simulink model "Boeing787_NewMission_ElectricalThermalHydraulicECS"  (R2016a)
settings: Solver=ode23tb  SolverMode=SingleTasking  StartTime=0.0  StopTime=346  RelTol=1e-3
InitFcn:
  | load('SampleOutput.mat')
  | 
  | load('SampleFuelBurn.mat')
undefined symbols (not defined in the file): ailerons, AirProp, B_737, CurrentMission, elevator, FuelBurn, HydProp, landing_gear, rudder, seed, thrust_rev
libraries: PowerFlowLib x68, simulink x20, powerlib_meascontrol x1
(part 15 of 24)

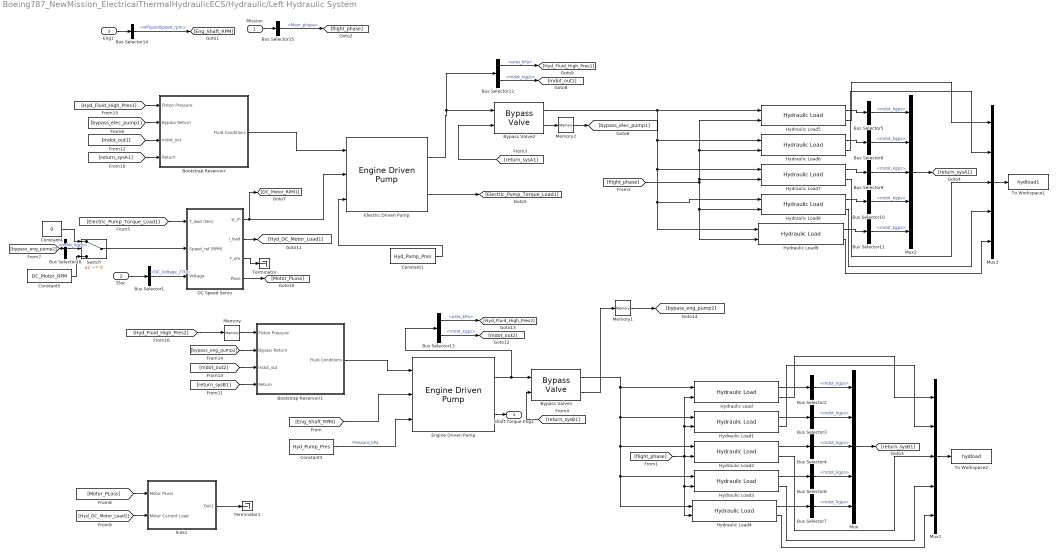
== system Boeing787_NewMission_ElectricalThermalHydraulicECS/Hydraulic/Left Hydraulic System ==
  Mission : Inport
  Elec : Inport  Port=2
  Eng1 : Inport  Port=3
  Bootstrap Reservoir : Subsystem  mask(Fluid Reservoir){res_vol=.25, High_Pres_Area=.05, Low_Pres_Area=0, pres_loss=1, T_init=300, P_init=1500, mass_init=30}
      mask prompts: res_vol "Resevoir Volume [m³]"; High_Pres_Area "High Pressure Piston Area"; Low_Pres_Area "Low Pressure Piston Area"; pres_loss "Air Pressure Losses [%]"; T_init "Initial Fluid Temp [K]"; P_init "Initial Air Pressure [kPa]"; mass_init "Initial Fluid Mass [kg]"
      mask help:
      | The fluid reservoir serves as a tank for storing excess hydraulic fluid.
      | The reservoir is fed by returning hydraulic fluid and feeds the engine driven pump.
      | Currently the fluid reservoir tracks the time dependent mass and temperature of the hydraulic fluid in the tank.
      |
      | Block Inputs
      | #1: Bleed air properties (Bus signal)
      | #2: Bypass return from bypass valve
      | #3: Mass flow rate pumped out by hydraulic pump
      | #4: Mass flow rate returned from actuators
      |
      | Block Outputs
      | #1: Bleed air demanded to maintain pressurization
      | #2: Hydraulic fluid properties in the reservoir
      mask init:
      | load AirProp
      | load HydProp
      mask Help: eval('open(''FluidReservoir_help.html'')');
      mask Display:
      | image(imread('hyd_res.png'))
      | 
      | port_label('input',1,'{\bf High Piston Pressure}','TexMode','on')
      | port_label('input',2,'{\bf Bypass Return}','TexMode','on')
      | port_label('input',3,'{\bf m_d_o_t Out}','TexMode','on')
      | port_label('input',4,'{\bf m_d_o_t Return}','TexMode','on')
      | 
      | 
      | port_label('output',1,'{\bf Fluid Out}','TexMode','on')
  Bootstrap Reservoir1 : Subsystem  mask(Fluid Reservoir){res_vol=.25, High_Pres_Area=.05, Low_Pres_Area=0, pres_loss=1, T_init=300, P_init=1500, mass_init=30}
      mask prompts: res_vol "Resevoir Volume [m³]"; High_Pres_Area "High Pressure Piston Area"; Low_Pres_Area "Low Pressure Piston Area"; pres_loss "Air Pressure Losses [%]"; T_init "Initial Fluid Temp [K]"; P_init "Initial Air Pressure [kPa]"; mass_init "Initial Fluid Mass [kg]"
      mask help:
      | The fluid reservoir serves as a tank for storing excess hydraulic fluid.
      | The reservoir is fed by returning hydraulic fluid and feeds the engine driven pump.
      | Currently the fluid reservoir tracks the time dependent mass and temperature of the hydraulic fluid in the tank.
      |
      | Block Inputs
      | #1: Bleed air properties (Bus signal)
      | #2: Bypass return from bypass valve
      | #3: Mass flow rate pumped out by hydraulic pump
      | #4: Mass flow rate returned from actuators
      |
      | Block Outputs
      | #1: Bleed air demanded to maintain pressurization
      | #2: Hydraulic fluid properties in the reservoir
      mask init:
      | load AirProp
      | load HydProp
      mask Help: eval('open(''FluidReservoir_help.html'')');
      mask Display:
      | image(imread('hyd_res.png'))
      | 
      | port_label('input',1,'{\bf High Piston Pressure}','TexMode','on')
      | port_label('input',2,'{\bf Bypass Return}','TexMode','on')
      | port_label('input',3,'{\bf m_d_o_t Out}','TexMode','on')
      | port_label('input',4,'{\bf m_d_o_t Return}','TexMode','on')
      | 
      | 
      | port_label('output',1,'{\bf Fluid Out}','TexMode','on')
  Bus Selector1 : BusSelector  OutputSignals=signal1.DC_Voltage_270
  Bus Selector{2..11,16} (11 alike) : BusSelector  OutputSignals=mdot_kgps
  Bus Selector12 : BusSelector  OutputSignals=pres_kPa,mdot_kgps
  Bus Selector13 : BusSelector  OutputSignals=pres_kPa,mdot_kgps
  Bus Selector14 : BusSelector  OutputSignals=Spools.HPSpoolSpeed_rpm
  Bus Selector15 : BusSelector  OutputSignals=Mssn_phase
  Bypass Valve1 : PowerFlowLib/Energy & Power Systems/Hydraulic/Bypass Valve
  Bypass Valve2 : PowerFlowLib/Energy & Power Systems/Hydraulic/Bypass Valve
  Constant1 : Constant  Value=Hyd_Pump_Pres
  Constant3 : Constant  Value=Hyd_Pump_Pres
  Constant4 : Constant  Value=0
  Constant5 : Constant  Value=DC_Motor_RPM
  DC Speed Servo : Subsystem  AncestorBlock=PowerFlowLib/Energy & Power Systems/Electrical/Machines/DC Speed Servo  mask{Vf=280, Ra=0.05, La=0.9e-3, Rfsh=400, Lfsh=320, Lmsh=1.9, J=1.5}
      mask prompts: Vf "Field voltage (V)"; Ra "Armature resistance (Ohms)"; La "Armature inductance (H)"; Rfsh "Shunt field resistance (Ohms)"; Lfsh "Shunt field inductance (H)"; Lmsh "Mutual inductance (H)"; J "Rotor moment of inertia (Kgm^2)"
  Electric Driven Pump : PowerFlowLib/Energy & Power Systems/Hydraulic/Engine Driven Pump  RPM=3750  disp=39  eta_mech=95  eta_v=85  nom_T=40  nom_w=393  nom_delP=20684
  Engine Driven Pump : PowerFlowLib/Energy & Power Systems/Hydraulic/Engine Driven Pump  RPM=3750  disp=39  eta_mech=95  eta_v=85  nom_T=40  nom_w=393  nom_delP=20684
  Hydraulic Load : PowerFlowLib/Energy & Power Systems/Hydraulic/Hydraulic Load  fileslct=off  filename=HydraulicLoad.mat  filedir=C:\Users\mwillms4\Dropbox\School\Graduate\Research\PowerFlow Development\PowerFlow Summer 2013\PropertyTables\HydraulicLoad.mat  var_struct=HydraulicLoad  h_load=B_737 - rudder
  Hydraulic Load1 : PowerFlowLib/Energy & Power Systems/Hydraulic/Hydraulic Load  fileslct=off  filename=HydraulicLoad.mat  filedir=C:\Users\mwillms4\Dropbox\School\Graduate\Research\PowerFlow Development\PowerFlow Summer 2013\PropertyTables\HydraulicLoad.mat  var_struct=HydraulicLoad  h_load=B_737 - ailerons
  Hydraulic Load2 : PowerFlowLib/Energy & Power Systems/Hydraulic/Hydraulic Load  fileslct=off  filename=HydraulicLoad.mat  filedir=C:\Users\mwillms4\Dropbox\School\Graduate\Research\PowerFlow Development\PowerFlow Summer 2013\PropertyTables\HydraulicLoad.mat  var_struct=HydraulicLoad  h_load=B_737 - elevator
  Hydraulic Load3 : PowerFlowLib/Energy & Power Systems/Hydraulic/Hydraulic Load  fileslct=off  filename=HydraulicLoad.mat  filedir=C:\Users\mwillms4\Dropbox\School\Graduate\Research\PowerFlow Development\PowerFlow Summer 2013\PropertyTables\HydraulicLoad.mat  var_struct=HydraulicLoad  h_load=B_737 - landing_gear
  Hydraulic Load4 : PowerFlowLib/Energy & Power Systems/Hydraulic/Hydraulic Load  fileslct=off  filename=HydraulicLoad.mat  filedir=C:\Users\mwillms4\Dropbox\School\Graduate\Research\PowerFlow Development\PowerFlow Summer 2013\PropertyTables\HydraulicLoad.mat  var_struct=HydraulicLoad  h_load=B_737 - thrust_rev
  Hydraulic Load5 : PowerFlowLib/Energy & Power Systems/Hydraulic/Hydraulic Load  fileslct=off  filename=HydraulicLoad.mat  filedir=C:\Users\mwillms4\Dropbox\School\Graduate\Research\PowerFlow Development\PowerFlow Summer 2013\PropertyTables\HydraulicLoad.mat  var_struct=HydraulicLoad  h_load=B_737 - rudder
  Hydraulic Load6 : PowerFlowLib/Energy & Power Systems/Hydraulic/Hydraulic Load  fileslct=off  filename=HydraulicLoad.mat  filedir=C:\Users\mwillms4\Dropbox\School\Graduate\Research\PowerFlow Development\PowerFlow Summer 2013\PropertyTables\HydraulicLoad.mat  var_struct=HydraulicLoad  h_load=B_737 - ailerons
  Hydraulic Load7 : PowerFlowLib/Energy & Power Systems/Hydraulic/Hydraulic Load  fileslct=off  filename=HydraulicLoad.mat  filedir=C:\Users\mwillms4\Dropbox\School\Graduate\Research\PowerFlow Development\PowerFlow Summer 2013\PropertyTables\HydraulicLoad.mat  var_struct=HydraulicLoad  h_load=B_737 - elevator
  Hydraulic Load8 : PowerFlowLib/Energy & Power Systems/Hydraulic/Hydraulic Load  fileslct=off  filename=HydraulicLoad.mat  filedir=C:\Users\mwillms4\Dropbox\School\Graduate\Research\PowerFlow Development\PowerFlow Summer 2013\PropertyTables\HydraulicLoad.mat  var_struct=HydraulicLoad  h_load=B_737 - landing_gear
  Hydraulic Load9 : PowerFlowLib/Energy & Power Systems/Hydraulic/Hydraulic Load  fileslct=off  filename=HydraulicLoad.mat  filedir=C:\Users\mwillms4\Dropbox\School\Graduate\Research\PowerFlow Development\PowerFlow Summer 2013\PropertyTables\HydraulicLoad.mat  var_struct=HydraulicLoad  h_load=B_737 - thrust_rev
  Memory : Memory
  Memory1 : Memory
  Memory2 : Memory
  Mux{,1..3} (4 alike) : Mux  Inputs=5
  Sinks : Subsystem
  Switch : Switch  Criteria=u2 ~= 0
  Terminator : Terminator
  Terminator1 : Terminator
  To Workspace1 : ToWorkspace  VariableName=hydload1  SaveFormat=Structure With Time  SampleTime=10
  To Workspace2 : ToWorkspace  VariableName=hydload  SaveFormat=Structure With Time  SampleTime=10
  Shaft Torque Eng1 : Outport
  wires:
  Bus Selector15/1 -> [flight_phase]  "<Mssn_phase>"
  Mission/1 -> Bus Selector15/1
  DC Speed Servo/1(w_m) -> Electric Driven Pump/2, [DC_Motor_RPM1]
  Constant3/1 -> Engine Driven Pump/3  "Pressure_kPa"
  Eng1/1 -> Bus Selector14/1
  [Eng_Shaft_RPM] -> Engine Driven Pump/2
  Elec/1 -> Bus Selector1/1
  Bus Selector1/1 -> DC Speed Servo/3(Voltage)  "<DC_Voltage_270>"
  Engine Driven Pump/2 -> Shaft Torque Eng1/1
  Hydraulic Load/1 -> Bus Selector2/1
  Bypass Valve1/1 -> Hydraulic Load3/1, Hydraulic Load4/1, Hydraulic Load2/1, Hydraulic Load1/1, Hydraulic Load/1
  Hydraulic Load1/2 -> Mux1/2
  Hydraulic Load2/2 -> Mux1/3
  Hydraulic Load1/1 -> Bus Selector3/1
  Hydraulic Load2/1 -> Bus Selector4/1
  Bus Selector3/1 -> Mux/2  "<mdot_kgps>"
  Bus Selector2/1 -> Mux/1  "<mdot_kgps>"
  Bus Selector4/1 -> Mux/3  "<mdot_kgps>"
  Mux/1 -> [return_sysB1]
  [flight_phase] -> Hydraulic Load/2, Hydraulic Load1/2, Hydraulic Load3/2, Hydraulic Load4/2, Hydraulic Load2/2
  Hydraulic Load3/1 -> Bus Selector6/1
  Hydraulic Load4/1 -> Bus Selector7/1
  Hydraulic Load4/2 -> Mux1/5
  Hydraulic Load3/2 -> Mux1/4
  Bus Selector6/1 -> Mux/4  "<mdot_kgps>"
  Bus Selector7/1 -> Mux/5  "<mdot_kgps>"
  Hydraulic Load/2 -> Mux1/1
  Mux1/1 -> To Workspace2/1
  Hydraulic Load5/1 -> Bus Selector5/1
  Bypass Valve2/1 -> Hydraulic Load9/1, Hydraulic Load8/1, Hydraulic Load7/1, Hydraulic Load6/1, Hydraulic Load5/1
  Hydraulic Load6/2 -> Mux3/2
  Hydraulic Load7/2 -> Mux3/3
  Hydraulic Load6/1 -> Bus Selector8/1
  Hydraulic Load7/1 -> Bus Selector9/1
  Bus Selector8/1 -> Mux2/2  "<mdot_kgps>"
  Bus Selector5/1 -> Mux2/1  "<mdot_kgps>"
  Bus Selector9/1 -> Mux2/3  "<mdot_kgps>"
  Mux2/1 -> [return_sysA1]
  [flight_phase] -> Hydraulic Load9/2, Hydraulic Load8/2, Hydraulic Load5/2, Hydraulic Load6/2, Hydraulic Load7/2
  Hydraulic Load8/1 -> Bus Selector10/1
  Hydraulic Load9/1 -> Bus Selector11/1
  Hydraulic Load9/2 -> Mux3/5
  Hydraulic Load8/2 -> Mux3/4
  Bus Selector10/1 -> Mux2/4  "<mdot_kgps>"
  Bus Selector11/1 -> Mux2/5  "<mdot_kgps>"
  Hydraulic Load5/2 -> Mux3/1
  Mux3/1 -> To Workspace1/1
  Engine Driven Pump/1 -> Bus Selector13/1, Bypass Valve1/1
  Electric Driven Pump/1 -> Bus Selector12/1, Bypass Valve2/1
  [return_sysA1] -> Bypass Valve2/2
  [return_sysB1] -> Bypass Valve1/2
  Constant1/1 -> Electric Driven Pump/3
  Electric Driven Pump/2 -> [Electric_Pump_Torque_Load1]
  [Electric_Pump_Torque_Load1] -> DC Speed Servo/1(T_load (Nm))
  Bypass Valve2/2 -> Memory2/1
  [bypass_elec_pump1] -> Bootstrap Reservoir/2(Bypass Return)
  Bootstrap Reservoir/1(Fluid Conditions) -> Electric Driven Pump/1
  Constant4/1 -> Switch/1
  Bus Selector12/1 -> [Hyd_Fluid_High_Pres1]  "<pres_kPa>"
  Bus Selector12/2 -> [mdot_out1]  "<mdot_kgps>"
  DC Speed Servo/4(Ploss) -> [Motor_PLoss]
  [Motor_PLoss] -> Sinks/1("Motor PLoss ")
  DC Speed Servo/2(i_load) -> [Hyd_DC_Motor_Load1]
  [Hyd_DC_Motor_Load1] -> Sinks/2(Motor Current Load)
  Bootstrap Reservoir1/1(Fluid Conditions) -> Engine Driven Pump/1
  Bus Selector13/1 -> [Hyd_Fluid_High_Pres2]  "<pres_kPa>"
  Bus Selector13/2 -> [mdot_out2]  "<mdot_kgps>"
  [return_sysA1] -> Bootstrap Reservoir/4(Return)
  [return_sysB1] -> Bootstrap Reservoir1/4(Return)
  [mdot_out1] -> Bootstrap Reservoir/3(mdot_out)
  Bypass Valve1/2 -> Memory1/1
  [bypass_eng_pump2] -> Bootstrap Reservoir1/2(Bypass Return)
  [mdot_out2] -> Bootstrap Reservoir1/3(mdot_out)
  [Hyd_Fluid_High_Pres1] -> Bootstrap Reservoir/1(Piston Pressure)
  [Hyd_Fluid_High_Pres2] -> Memory/1
  Bus Selector14/1 -> [Eng_Shaft_RPM]  "<HPSpoolSpeed_rpm>"
  DC Speed Servo/3(T_em) -> Terminator/1
  Sinks/1(Out1) -> Terminator1/1
  Memory/1 -> Bootstrap Reservoir1/1(Piston Pressure)
  [bypass_eng_pump2] -> Bus Selector16/1
  Constant5/1 -> Switch/3
  Bus Selector16/1 -> Switch/2  "<mdot_kgps>"
  Switch/1 -> DC Speed Servo/2(Speed_ref (RPM))
  Memory1/1 -> [bypass_eng_pump2]
  Memory2/1 -> [bypass_elec_pump1]

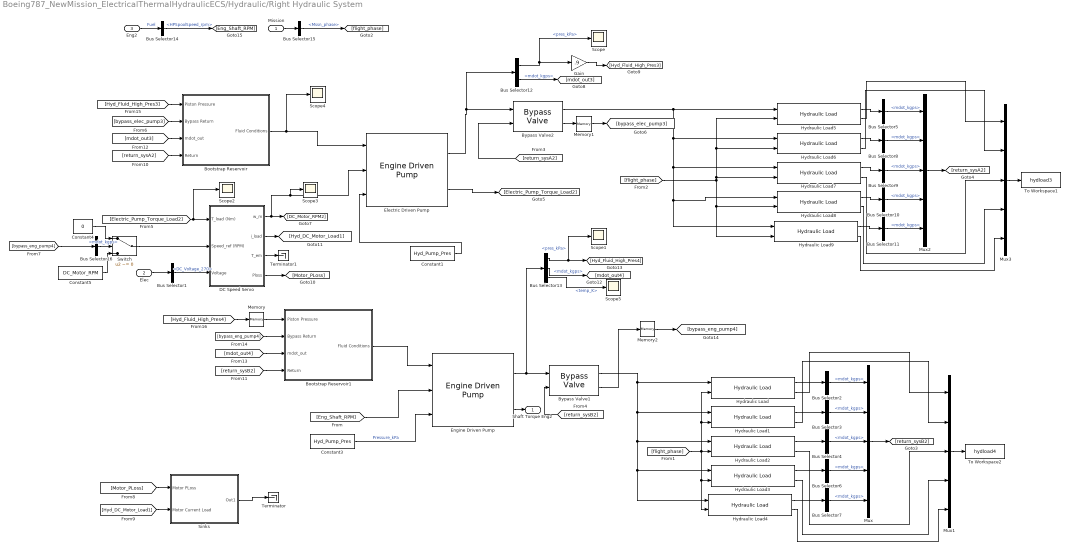
== system Boeing787_NewMission_ElectricalThermalHydraulicECS/Hydraulic/Right Hydraulic System ==
  Mission : Inport
  Elec : Inport  Port=2
  Eng2 : Inport  Port=3
  Bootstrap Reservoir : Subsystem  mask(Fluid Reservoir){res_vol=.25, High_Pres_Area=.05, Low_Pres_Area=0, pres_loss=1, T_init=300, P_init=1500, mass_init=30}
      mask prompts: res_vol "Resevoir Volume [m³]"; High_Pres_Area "High Pressure Piston Area"; Low_Pres_Area "Low Pressure Piston Area"; pres_loss "Air Pressure Losses [%]"; T_init "Initial Fluid Temp [K]"; P_init "Initial Air Pressure [kPa]"; mass_init "Initial Fluid Mass [kg]"
      mask help:
      | The fluid reservoir serves as a tank for storing excess hydraulic fluid.
      | The reservoir is fed by returning hydraulic fluid and feeds the engine driven pump.
      | Currently the fluid reservoir tracks the time dependent mass and temperature of the hydraulic fluid in the tank.
      |
      | Block Inputs
      | #1: Bleed air properties (Bus signal)
      | #2: Bypass return from bypass valve
      | #3: Mass flow rate pumped out by hydraulic pump
      | #4: Mass flow rate returned from actuators
      |
      | Block Outputs
      | #1: Bleed air demanded to maintain pressurization
      | #2: Hydraulic fluid properties in the reservoir
      mask init:
      | load AirProp
      | load HydProp
      mask Help: eval('open(''FluidReservoir_help.html'')');
      mask Display:
      | image(imread('hyd_res.png'))
      | 
      | port_label('input',1,'{\bf High Piston Pressure}','TexMode','on')
      | port_label('input',2,'{\bf Bypass Return}','TexMode','on')
      | port_label('input',3,'{\bf m_d_o_t Out}','TexMode','on')
      | port_label('input',4,'{\bf m_d_o_t Return}','TexMode','on')
      | 
      | 
      | port_label('output',1,'{\bf Fluid Out}','TexMode','on')
  Bootstrap Reservoir1 : Subsystem  mask(Fluid Reservoir){res_vol=.25, High_Pres_Area=.05, Low_Pres_Area=0, pres_loss=1, T_init=300, P_init=1500, mass_init=30}
      mask prompts: res_vol "Resevoir Volume [m³]"; High_Pres_Area "High Pressure Piston Area"; Low_Pres_Area "Low Pressure Piston Area"; pres_loss "Air Pressure Losses [%]"; T_init "Initial Fluid Temp [K]"; P_init "Initial Air Pressure [kPa]"; mass_init "Initial Fluid Mass [kg]"
      mask help:
      | The fluid reservoir serves as a tank for storing excess hydraulic fluid.
      | The reservoir is fed by returning hydraulic fluid and feeds the engine driven pump.
      | Currently the fluid reservoir tracks the time dependent mass and temperature of the hydraulic fluid in the tank.
      |
      | Block Inputs
      | #1: Bleed air properties (Bus signal)
      | #2: Bypass return from bypass valve
      | #3: Mass flow rate pumped out by hydraulic pump
      | #4: Mass flow rate returned from actuators
      |
      | Block Outputs
      | #1: Bleed air demanded to maintain pressurization
      | #2: Hydraulic fluid properties in the reservoir
      mask init:
      | load AirProp
      | load HydProp
      mask Help: eval('open(''FluidReservoir_help.html'')');
      mask Display:
      | image(imread('hyd_res.png'))
      | 
      | port_label('input',1,'{\bf High Piston Pressure}','TexMode','on')
      | port_label('input',2,'{\bf Bypass Return}','TexMode','on')
      | port_label('input',3,'{\bf m_d_o_t Out}','TexMode','on')
      | port_label('input',4,'{\bf m_d_o_t Return}','TexMode','on')
      | 
      | 
      | port_label('output',1,'{\bf Fluid Out}','TexMode','on')
  Bus Selector1 : BusSelector  OutputSignals=signal1.DC_Voltage_270
  Bus Selector{2..11,16} (11 alike) : BusSelector  OutputSignals=mdot_kgps
  Bus Selector12 : BusSelector  OutputSignals=pres_kPa,mdot_kgps
  Bus Selector13 : BusSelector  OutputSignals=pres_kPa,mdot_kgps,temp_K
  Bus Selector14 : BusSelector  OutputSignals=Spools.HPSpoolSpeed_rpm
  Bus Selector15 : BusSelector  OutputSignals=Mssn_phase
  Bypass Valve1 : PowerFlowLib/Energy & Power Systems/Hydraulic/Bypass Valve
  Bypass Valve2 : PowerFlowLib/Energy & Power Systems/Hydraulic/Bypass Valve
  Constant1 : Constant  Value=Hyd_Pump_Pres
  Constant3 : Constant  Value=Hyd_Pump_Pres
  Constant4 : Constant  Value=0
  Constant5 : Constant  Value=DC_Motor_RPM
  DC Speed Servo : Subsystem  AncestorBlock=PowerFlowLib/Energy & Power Systems/Electrical/Machines/DC Speed Servo  mask{Vf=390, Ra=0.05, La=0.9e-3, Rfsh=400, Lfsh=320, Lmsh=1.9, J=1.5}
      mask prompts: Vf "Field voltage (V)"; Ra "Armature resistance (Ohms)"; La "Armature inductance (H)"; Rfsh "Shunt field resistance (Ohms)"; Lfsh "Shunt field inductance (H)"; Lmsh "Mutual inductance (H)"; J "Rotor moment of inertia (Kgm^2)"
  Electric Driven Pump : PowerFlowLib/Energy & Power Systems/Hydraulic/Engine Driven Pump  RPM=3750  disp=39  eta_mech=95  eta_v=85  nom_T=40  nom_w=393  nom_delP=20684
  Engine Driven Pump : PowerFlowLib/Energy & Power Systems/Hydraulic/Engine Driven Pump  RPM=3750  disp=39  eta_mech=95  eta_v=85  nom_T=40  nom_w=393  nom_delP=20684
  Gain : Gain  Gain=.9
  Hydraulic Load : PowerFlowLib/Energy & Power Systems/Hydraulic/Hydraulic Load  fileslct=off  filename=HydraulicLoad.mat  filedir=C:\Users\mwillms4\Dropbox\School\Graduate\Research\PowerFlow Development\PowerFlow Summer 2013\PropertyTables\HydraulicLoad.mat  var_struct=HydraulicLoad  h_load=B_737 - rudder
  Hydraulic Load1 : PowerFlowLib/Energy & Power Systems/Hydraulic/Hydraulic Load  fileslct=off  filename=HydraulicLoad.mat  filedir=C:\Users\mwillms4\Dropbox\School\Graduate\Research\PowerFlow Development\PowerFlow Summer 2013\PropertyTables\HydraulicLoad.mat  var_struct=HydraulicLoad  h_load=B_737 - ailerons
  Hydraulic Load2 : PowerFlowLib/Energy & Power Systems/Hydraulic/Hydraulic Load  fileslct=off  filename=HydraulicLoad.mat  filedir=C:\Users\mwillms4\Dropbox\School\Graduate\Research\PowerFlow Development\PowerFlow Summer 2013\PropertyTables\HydraulicLoad.mat  var_struct=HydraulicLoad  h_load=B_737 - elevator
  Hydraulic Load3 : PowerFlowLib/Energy & Power Systems/Hydraulic/Hydraulic Load  fileslct=off  filename=HydraulicLoad.mat  filedir=C:\Users\mwillms4\Dropbox\School\Graduate\Research\PowerFlow Development\PowerFlow Summer 2013\PropertyTables\HydraulicLoad.mat  var_struct=HydraulicLoad  h_load=B_737 - landing_gear
  Hydraulic Load4 : PowerFlowLib/Energy & Power Systems/Hydraulic/Hydraulic Load  fileslct=off  filename=HydraulicLoad.mat  filedir=C:\Users\mwillms4\Dropbox\School\Graduate\Research\PowerFlow Development\PowerFlow Summer 2013\PropertyTables\HydraulicLoad.mat  var_struct=HydraulicLoad  h_load=B_737 - thrust_rev
  Hydraulic Load5 : PowerFlowLib/Energy & Power Systems/Hydraulic/Hydraulic Load  fileslct=off  filename=HydraulicLoad.mat  filedir=C:\Users\mwillms4\Dropbox\School\Graduate\Research\PowerFlow Development\PowerFlow Summer 2013\PropertyTables\HydraulicLoad.mat  var_struct=HydraulicLoad  h_load=B_737 - rudder
  Hydraulic Load6 : PowerFlowLib/Energy & Power Systems/Hydraulic/Hydraulic Load  fileslct=off  filename=HydraulicLoad.mat  filedir=C:\Users\mwillms4\Dropbox\School\Graduate\Research\PowerFlow Development\PowerFlow Summer 2013\PropertyTables\HydraulicLoad.mat  var_struct=HydraulicLoad  h_load=B_737 - ailerons
  Hydraulic Load7 : PowerFlowLib/Energy & Power Systems/Hydraulic/Hydraulic Load  fileslct=off  filename=HydraulicLoad.mat  filedir=C:\Users\mwillms4\Dropbox\School\Graduate\Research\PowerFlow Development\PowerFlow Summer 2013\PropertyTables\HydraulicLoad.mat  var_struct=HydraulicLoad  h_load=B_737 - elevator
  Hydraulic Load8 : PowerFlowLib/Energy & Power Systems/Hydraulic/Hydraulic Load  fileslct=off  filename=HydraulicLoad.mat  filedir=C:\Users\mwillms4\Dropbox\School\Graduate\Research\PowerFlow Development\PowerFlow Summer 2013\PropertyTables\HydraulicLoad.mat  var_struct=HydraulicLoad  h_load=B_737 - landing_gear
  Hydraulic Load9 : PowerFlowLib/Energy & Power Systems/Hydraulic/Hydraulic Load  fileslct=off  filename=HydraulicLoad.mat  filedir=C:\Users\mwillms4\Dropbox\School\Graduate\Research\PowerFlow Development\PowerFlow Summer 2013\PropertyTables\HydraulicLoad.mat  var_struct=HydraulicLoad  h_load=B_737 - thrust_rev
  Memory : Memory
  Memory1 : Memory
  Memory2 : Memory
  Mux{,1..3} (4 alike) : Mux  Inputs=5
  Scope{,1..5} (6 alike) : Scope
  Sinks : Subsystem
  Switch : Switch  Criteria=u2 ~= 0
  Terminator : Terminator
  Terminator1 : Terminator
  To Workspace1 : ToWorkspace  VariableName=hydload3  SaveFormat=Structure With Time  SampleTime=10
  To Workspace2 : ToWorkspace  VariableName=hydload4  SaveFormat=Structure With Time  SampleTime=10
  Shaft Torque Eng2 : Outport
  wires:
  Bus Selector15/1 -> [flight_phase]  "<Mssn_phase>"
  Mission/1 -> Bus Selector15/1
  Constant3/1 -> Engine Driven Pump/3  "Pressure_kPa"
  [Eng_Shaft_RPM] -> Engine Driven Pump/2
  Elec/1 -> Bus Selector1/1
  Bus Selector1/1 -> DC Speed Servo/3(Voltage)  "<DC_Voltage_270>"
  Engine Driven Pump/2 -> Shaft Torque Eng2/1
  Hydraulic Load/1 -> Bus Selector2/1
  Bypass Valve1/1 -> Hydraulic Load3/1, Hydraulic Load4/1, Hydraulic Load2/1, Hydraulic Load1/1, Hydraulic Load/1
  Hydraulic Load1/2 -> Mux1/2
  Hydraulic Load2/2 -> Mux1/3
  Hydraulic Load1/1 -> Bus Selector3/1
  Hydraulic Load2/1 -> Bus Selector4/1
  Bus Selector3/1 -> Mux/2  "<mdot_kgps>"
  Bus Selector2/1 -> Mux/1  "<mdot_kgps>"
  Bus Selector4/1 -> Mux/3  "<mdot_kgps>"
  Mux/1 -> [return_sysB2]
  [flight_phase] -> Hydraulic Load/2, Hydraulic Load1/2, Hydraulic Load3/2, Hydraulic Load4/2, Hydraulic Load2/2
  Hydraulic Load3/1 -> Bus Selector6/1
  Hydraulic Load4/1 -> Bus Selector7/1
  Hydraulic Load4/2 -> Mux1/5
  Hydraulic Load3/2 -> Mux1/4
  Bus Selector6/1 -> Mux/4  "<mdot_kgps>"
  Bus Selector7/1 -> Mux/5  "<mdot_kgps>"
  Hydraulic Load/2 -> Mux1/1
  Mux1/1 -> To Workspace2/1
  Hydraulic Load5/1 -> Bus Selector5/1
  Bypass Valve2/1 -> Hydraulic Load9/1, Hydraulic Load8/1, Hydraulic Load7/1, Hydraulic Load6/1, Hydraulic Load5/1
  Hydraulic Load6/2 -> Mux3/2
  Hydraulic Load7/2 -> Mux3/3
  Hydraulic Load6/1 -> Bus Selector8/1
  Hydraulic Load7/1 -> Bus Selector9/1
  Bus Selector8/1 -> Mux2/2  "<mdot_kgps>"
  Bus Selector5/1 -> Mux2/1  "<mdot_kgps>"
  Bus Selector9/1 -> Mux2/3  "<mdot_kgps>"
  Mux2/1 -> [return_sysA2]
  [flight_phase] -> Hydraulic Load9/2, Hydraulic Load8/2, Hydraulic Load5/2, Hydraulic Load6/2, Hydraulic Load7/2
  Hydraulic Load8/1 -> Bus Selector10/1
  Hydraulic Load9/1 -> Bus Selector11/1
  Hydraulic Load9/2 -> Mux3/5
  Hydraulic Load8/2 -> Mux3/4
  Bus Selector10/1 -> Mux2/4  "<mdot_kgps>"
  Bus Selector11/1 -> Mux2/5  "<mdot_kgps>"
  Hydraulic Load5/2 -> Mux3/1
  Mux3/1 -> To Workspace1/1
  Engine Driven Pump/1 -> Bus Selector13/1, Bypass Valve1/1
  Electric Driven Pump/1 -> Bus Selector12/1, Bypass Valve2/1
  [return_sysA2] -> Bypass Valve2/2
  [return_sysB2] -> Bypass Valve1/2
  Constant1/1 -> Electric Driven Pump/3
  Bypass Valve2/2 -> Memory1/1
  [bypass_elec_pump3] -> Bootstrap Reservoir/2(Bypass Return)
  Bootstrap Reservoir/1(Fluid Conditions) -> Scope4/1, Electric Driven Pump/1
  Bus Selector12/1 -> Gain/1, Scope/1  "<pres_kPa>"
  Bus Selector12/2 -> [mdot_out3]  "<mdot_kgps>"
  DC Speed Servo/4(Ploss) -> [Motor_PLoss]
  [Motor_PLoss] -> Sinks/1("Motor PLoss ")
  DC Speed Servo/2(i_load) -> [Hyd_DC_Motor_Load1]
  [Hyd_DC_Motor_Load1] -> Sinks/2(Motor Current Load)
  Bootstrap Reservoir1/1(Fluid Conditions) -> Engine Driven Pump/1
  Bus Selector13/1 -> Scope1/1, [Hyd_Fluid_High_Pres4]  "<pres_kPa>"
  Bus Selector13/2 -> [mdot_out4]  "<mdot_kgps>"
  [return_sysA2] -> Bootstrap Reservoir/4(Return)
  [return_sysB2] -> Bootstrap Reservoir1/4(Return)
  [mdot_out3] -> Bootstrap Reservoir/3(mdot_out)
  Bypass Valve1/2 -> Memory2/1
  [bypass_eng_pump4] -> Bootstrap Reservoir1/2(Bypass Return)
  [mdot_out4] -> Bootstrap Reservoir1/3(mdot_out)
  [Hyd_Fluid_High_Pres3] -> Bootstrap Reservoir/1(Piston Pressure)
  [Hyd_Fluid_High_Pres4] -> Memory/1
  DC Speed Servo/3(T_em) -> Terminator1/1
  Sinks/1(Out1) -> Terminator/1
  Electric Driven Pump/2 -> [Electric_Pump_Torque_Load2]
  Switch/1 -> DC Speed Servo/2(Speed_ref (RPM))
  [Electric_Pump_Torque_Load2] -> DC Speed Servo/1(T_load (Nm)), Scope2/1
  DC Speed Servo/1(w_m) -> Scope3/1, Electric Driven Pump/2, [DC_Motor_RPM2]
  Gain/1 -> [Hyd_Fluid_High_Pres3]
  Memory/1 -> Bootstrap Reservoir1/1(Piston Pressure)
  Constant4/1 -> Switch/1
  Constant5/1 -> Switch/3
  Bus Selector16/1 -> Switch/2  "<mdot_kgps>"
  [bypass_eng_pump4] -> Bus Selector16/1
  Eng2/1 -> Bus Selector14/1  "Fuel"
  Bus Selector14/1 -> [Eng_Shaft_RPM]  "<HPSpoolSpeed_rpm>"
  Memory1/1 -> [bypass_elec_pump3]
  Memory2/1 -> [bypass_eng_pump4]
  Bus Selector13/3 -> Scope5/1  "<temp_K>"

== system Boeing787_NewMission_ElectricalThermalHydraulicECS/ECS/Left Pack/Compressor ==
  note: Flow
  note: N
  note: eff
  In2 : Inport
  In4 : Inport  Port=2
  Add : Sum
  Bias : Bias  Bias=-1
  Bus Creator1 : BusCreator  Inputs=3
  Bus Selector : BusSelector  OutputSignals=pres_kPa
  Bus Selector1 : BusSelector  OutputSignals=mdot_kgps
  Bus Selector2 : BusSelector  OutputSignals=temp_K
  Cp(P,T)1 : Lookup_n-D  BreakpointsForDimension1=AirProp.P  BreakpointsForDimension2=AirProp.T  BreakpointsForDimension3=[1]  Table=AirProp.Cp_pt  RndMeth=Simplest  InputSameDT=on
  Divide1 : Product  Inputs=/**
  Divide2 : Product  Inputs=***
  Divide3 : Product  Inputs=**
  Divide4 : Product  Inputs=/*
  Divide5 : Product  Inputs=/**
  Gain1 : Gain  Gain=1000
  K to R : Gain  Gain=1.8
  Math Function : Math  Operator=pow  SaturateOnIntegerOverflow=on
  Pressure_ratio : Lookup_n-D  BreakpointsForDimension1=[20,25,30,35,40,45,50,55,60,65,70,75,80,85,90]  BreakpointsForDimension2=[1097,1316,1536,1756,1975,2195,2414]  Table=reshape([1.22,1.202,1.18,1.145,1.05,1,1,1,1,1,1,1,1,1,1,1.325,1.31,1.3,1.275,1.22,1.16,1,1,1,1,1,1,1,1,1,1.49,1.485,1.475,1.45,1.41,1.38,1.3,1.15,1,1,1,1,1,1,1,1.65,1.65,1.63,1.628,1.61,1.598,1.55,1.5,1.4,1.1,1,1,1,1,1,1.885,1.87,1.87,1.86,1.83,1.82,1.8,1.76,1.7,1.62,1.5,1,1,1,1,2.15,2.15,2.15,2.14,2.12,2.05,2.085,2.05,2.01,1.98,1.902,1.8,1,1,1,2.45,2.44,2.43,2.42,2.41,2.405,2.4,2.39,2.365,2.32,2.28,2.2,2.14,2.02,1.7],15,7)  RndMeth=Simplest  InputSameDT=on
  Reciprocal Sqrt : Sqrt  SaturateOnIntegerOverflow=on
  Scope1 : Scope
  Scope5 : Scope
  Table1 : Lookup_n-D  BreakpointsForDimension1=[20,25,30,35,40,45,50,55,60,65,70,75,80,85,90]  BreakpointsForDimension2=[1097,1316,1536,1756,1975,2195,2414]  Table=reshape([0.84396,0.83224,0.7928,0.70795,0.33,0.16,0.16,0.16,0.16,0.16,0.16,0.16,0.16,0.16,0.16,0.8265,0.8272,0.823,0.8075,0.709,0.5437,0.0850000000000002,0.0850000000000002,0.0850000000000002,0.0850000000000002,0.0850000000000002,0.0850000000000002,0.0850000000000002,0.0850000000000002,0.0850000000000002,0.6962,0.716699999999999,0.753,0.8086,0.8094,0.777,0.672,0.3705,0.0690000000000002,0.0690000000000002,0.0690000000000002,0.0690000000000002,0.0690000000000002,0.0690000000000002,0.0690000000000002,0.803,0.803,0.8122,0.81312,0.82042,0.822052,0.8045,0.755,0.654,0.192,0.0480000000000002,0.0480000000000002,0.0480000000000002,0.0480000000000002,0.0480000000000002,0.79155,0.8025,0.8025,0.806,0.81335,0.8144,0.8165,0.811,0.7775,0.7328,0.628,0.0080000000000004,0.0080000000000004,0.0080000000000004,0.0080000000000004,0.802,0.802,0.802,0.802,0.802,0.8112,0.80584,0.8112,0.81728,0.80648,0.77466,0.723,0.00180000000000019,0.00180000000000019,0.00180000000000019,0.81,0.81,0.81,0.81,0.81,0.81,0.81,0.81,0.81,0.81,0.8068,0.7888,0.766,0.72408,0.54796],15,7)  RndMeth=Simplest  InputSameDT=on
  "m and P " : Gain
  poly index : Constant  Value=(1.4-1)/1.4
  Out1 : Outport
  Power_out : Outport  Port=2
  wires:
  Gain1/1 -> Divide2/2
  Cp(P,T)1/1 -> Gain1/1
  In2/1 -> Bus Selector/1, Bus Selector1/1, Bus Selector2/1
  Bus Selector2/1 -> Divide1/3, Add/2, K to R/1  "<temp_K>"
  Reciprocal Sqrt/1 -> Divide4/1, Divide5/3
  Bus Selector1/1 -> Divide2/1, Bus Creator1/2, Divide5/2  "<mdot_kgps>"
  Pressure_ratio/1 -> Math Function/1, Divide3/2
  poly index/1 -> Math Function/2
  Math Function/1 -> Bias/1
  Bias/1 -> Divide1/2
  Divide1/1 -> Cp(P,T)1/2, Divide2/3, Add/1
  Divide2/1 -> Power_out/1
  Bus Selector/1 -> Divide3/1, Divide5/1  "<pres_kPa>"
  Divide3/1 -> Cp(P,T)1/1, Bus Creator1/1  "pres_kPa"
  Add/1 -> Bus Creator1/3  "temp_K"
  Bus Creator1/1 -> Out1/1
  K to R/1 -> Reciprocal Sqrt/1
  In4/1 -> Scope1/1, Divide4/2
  Divide4/1 -> Scope5/1, Pressure_ratio/2, Table1/2
  Divide5/1 -> "m and P "/1
  "m and P "/1 -> Pressure_ratio/1, Table1/1
  Table1/1 -> Divide1/1

== system Boeing787_NewMission_ElectricalThermalHydraulicECS/ECS/Left Pack/DC Speed Servo1 ==
  T_load (Nm) : Inport
  Speed_ref (RPM) : Inport  Port=2
  Voltage : Inport  Port=3
  DC Machine : Subsystem
  Fcn : Fcn  Expr=u(1)/(u(2)+0.1)
  Gain2 : Gain  Gain=60/(2*pi)
  Mux : Mux  Inputs=2
  PID Controller : simulink/Continuous/PID Controller  Controller=PID  TimeDomain=Continuous-time  SampleTime=-1  IntegratorMethod=Forward Euler  FilterMethod=Forward Euler  Form=Parallel  UseFilter=on  ControllerParametersSource=internal  P=1  I=0.1  D=0  N=100  InitialConditionSource=internal  InitialConditionForIntegrator=0  InitialConditionForFilter=0  ExternalReset=none  LimitOutput=off  UpperSaturationLimit=inf  LowerSaturationLimit=-inf  LinearizeAsGain=on  AntiWindupMode=none  Kb=1  TrackingMode=off  Kt=1  PParamMin=[]  PParamMax=[]  IParamMin=[]  IParamMax=[]  DParamMin=[]  DParamMax=[]  NParamMin=[]  NParamMax=[]  KbParamMin=[]  KbParamMax=[]  KtParamMin=[]  KtParamMax=[]  POutMin=[]  POutMax=[]  IOutMin=[]  IOutMax=[]  DOutMin=[]  DOutMax=[]  NOutMin=[]  NOutMax=[]  KbOutMin=[]  KbOutMax=[]  KtOutMin=[]  KtOutMax=[]  IntegratorOutMin=[]  IntegratorOutMax=[]  FilterOutMin=[]  FilterOutMax=[]  SumOutMin=[]  SumOutMax=[]  SumI1OutMin=[]  SumI1OutMax=[]  SumI2OutMin=[]  SumI2OutMax=[]  SumI3OutMin=[]  SumI3OutMax=[]  SumDOutMin=[]  SumDOutMax=[]  SaturationOutMin=[]  SaturationOutMax=[]  IntegratorContinuousStateAttributes=''  IntegratorStateMustResolveToSignalObject=off  IntegratorRTWStateStorageClass=Auto  FilterContinuousStateAttributes=''  FilterStateMustResolveToSignalObject=off  FilterRTWStateStorageClass=Auto  DifferentiatorICPrevScaledInput=0  DifferentiatorOutMin=[]  DifferentiatorOutMax=[]
  Sum : Sum  Inputs=-+|
  Terminator{,1..3} (4 alike) : Terminator
  w_m : Outport
  i_load : Outport  Port=2
  T_em : Outport  Port=3
  Ploss : Outport  Port=4
  wires:
  DC Machine/5(Plosses) -> Ploss/1
  Sum/1 -> PID Controller/1
  Gain2/1 -> Sum/1, w_m/1
  Speed_ref (RPM)/1 -> Sum/2
  T_load (Nm)/1 -> DC Machine/3(Tload)
  DC Machine/6(Te) -> T_em/1
  Mux/1 -> Fcn/1
  DC Machine/3(Pe) -> Mux/1
  Fcn/1 -> i_load/1
  DC Machine/7(Speed) -> Gain2/1
  Voltage/1 -> DC Machine/1(Vf), Mux/2
  PID Controller/1 -> DC Machine/2(Va)
  DC Machine/1(If) -> Terminator/1
  DC Machine/2(Ia) -> Terminator1/1
  DC Machine/4(Pm) -> Terminator2/1
  DC Machine/8(theta) -> Terminator3/1

== system Boeing787_NewMission_ElectricalThermalHydraulicECS/ECS/Left Pack/DC Speed Servo2 ==
  T_load (Nm) : Inport
  Speed_ref (RPM) : Inport  Port=2
  Voltage : Inport  Port=3
  DC Machine : Subsystem
  Fcn : Fcn  Expr=u(1)/(u(2)+0.1)
  Gain2 : Gain  Gain=60/(2*pi)
  Mux : Mux  Inputs=2
  PID Controller : simulink/Continuous/PID Controller  Controller=PID  TimeDomain=Continuous-time  SampleTime=-1  IntegratorMethod=Forward Euler  FilterMethod=Forward Euler  Form=Parallel  UseFilter=on  ControllerParametersSource=internal  P=1  I=0.1  D=0  N=100  InitialConditionSource=internal  InitialConditionForIntegrator=0  InitialConditionForFilter=0  ExternalReset=none  LimitOutput=off  UpperSaturationLimit=inf  LowerSaturationLimit=-inf  LinearizeAsGain=on  AntiWindupMode=none  Kb=1  TrackingMode=off  Kt=1  PParamMin=[]  PParamMax=[]  IParamMin=[]  IParamMax=[]  DParamMin=[]  DParamMax=[]  NParamMin=[]  NParamMax=[]  KbParamMin=[]  KbParamMax=[]  KtParamMin=[]  KtParamMax=[]  POutMin=[]  POutMax=[]  IOutMin=[]  IOutMax=[]  DOutMin=[]  DOutMax=[]  NOutMin=[]  NOutMax=[]  KbOutMin=[]  KbOutMax=[]  KtOutMin=[]  KtOutMax=[]  IntegratorOutMin=[]  IntegratorOutMax=[]  FilterOutMin=[]  FilterOutMax=[]  SumOutMin=[]  SumOutMax=[]  SumI1OutMin=[]  SumI1OutMax=[]  SumI2OutMin=[]  SumI2OutMax=[]  SumI3OutMin=[]  SumI3OutMax=[]  SumDOutMin=[]  SumDOutMax=[]  SaturationOutMin=[]  SaturationOutMax=[]  IntegratorContinuousStateAttributes=''  IntegratorStateMustResolveToSignalObject=off  IntegratorRTWStateStorageClass=Auto  FilterContinuousStateAttributes=''  FilterStateMustResolveToSignalObject=off  FilterRTWStateStorageClass=Auto  DifferentiatorICPrevScaledInput=0  DifferentiatorOutMin=[]  DifferentiatorOutMax=[]
  Sum : Sum  Inputs=-+|
  Terminator{,1..3} (4 alike) : Terminator
  w_m : Outport
  i_load : Outport  Port=2
  T_em : Outport  Port=3
  Ploss : Outport  Port=4
  wires:
  DC Machine/5(Plosses) -> Ploss/1
  Sum/1 -> PID Controller/1
  Gain2/1 -> Sum/1, w_m/1
  Speed_ref (RPM)/1 -> Sum/2
  T_load (Nm)/1 -> DC Machine/3(Tload)
  DC Machine/6(Te) -> T_em/1
  Mux/1 -> Fcn/1
  DC Machine/3(Pe) -> Mux/1
  Fcn/1 -> i_load/1
  DC Machine/7(Speed) -> Gain2/1
  Voltage/1 -> DC Machine/1(Vf), Mux/2
  PID Controller/1 -> DC Machine/2(Va)
  DC Machine/1(If) -> Terminator/1
  DC Machine/2(Ia) -> Terminator1/1
  DC Machine/4(Pm) -> Terminator2/1
  DC Machine/8(theta) -> Terminator3/1

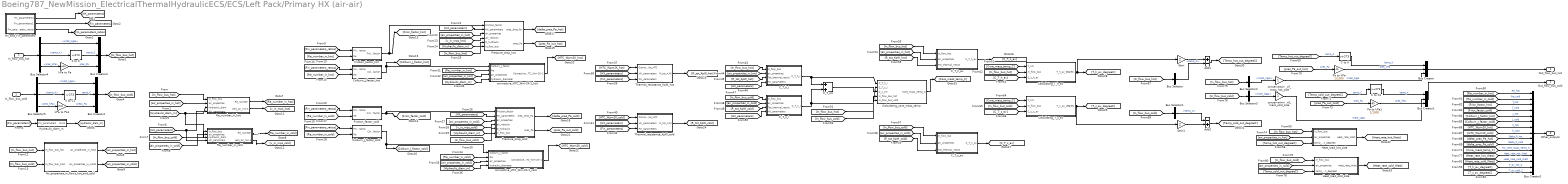
== system Boeing787_NewMission_ElectricalThermalHydraulicECS/ECS/Left Pack/Primary HX (air-air) ==
  In_flow_bus_hot : Inport
  In_flow_bus_cold : Inport  Port=2
  Add1 : Sum  Inputs=+-
  Add2 : Sum  Inputs=-+
  Air_properties_in_flows_hot_and_cold : Subsystem
  Bus Creator{,1,3..4} (4 alike) : BusCreator  Inputs=3
  Bus Creator2 : BusCreator  Inputs=15
  Bus Selector : BusSelector  OutputSignals=temp_C
  Bus Selector1 : BusSelector  OutputSignals=temp_C
  Bus Selector2 : BusSelector  OutputSignals=mdot_kgps
  Bus Selector3 : BusSelector  OutputSignals=mdot_kgps
  Bus Selector4 : BusSelector  OutputSignals=mdot_kgps,temp_K,pres_kPa
  Bus Selector5 : BusSelector  OutputSignals=mdot_kgps,temp_K,pres_kPa
  C to K : Bias  Bias=273
  C to K1 : Bias  Bias=273
  C_T_c_av : Subsystem
  C_T_c_i : Subsystem
  C_T_cm : Sum
  C_T_h_av : Subsystem
  C_T_h_i : Subsystem
  Calculating_T_c_av : Subsystem
  Calculating_T_h_av : Subsystem
  Calculating_core_mass_temp : Subsystem
  Colburn_J_factor_cold : Subsystem
  Colburn_J_factor_hot : Subsystem
  Friction_factor_cold : Subsystem
  Friction_factor_hot : Subsystem
  Gain : Gain  Gain=2
  Gain1 : Gain  Gain=2
  HX_and_Fin_paramters : Subsystem
  Heat_load_cold_side : Subsystem
  Heat_load_hot_side : Subsystem
  Hydraulic_diam_m : Subsystem
  K to C : Bias  Bias=-273
  K to C1 : Bias  Bias=-273
  Pa to kPa : Gain  Gain=1/1000
  Pa to kPa1 : Gain  Gain=1/1000
  Pressure_drop_cold : Subsystem
  Pressure_drop_hot : Subsystem
  Re_number_in_cold : Subsystem
  Re_number_in_hot : Subsystem
  Thermal_resistance_KpW_cold : Subsystem
  Thermal_resistance_KpW_hot : Subsystem
  conservation _of_mass_cold_side : Gain
  conservation _of_mass_hot_side : Gain
  convective_HTC_Wm-2K-1_cold : Subsystem
  convective_HTC_Wm-2K-1_hot : Subsystem
  kPa to Pa : Gain  Gain=1000
  kPa to Pa1 : Gain  Gain=1000
  Out_flow_bus_hot : Outport
  Out_flow_bus_cold : Outport  Port=2
  Other_outputs : Outport  Port=3
  wires:
  Heat_load_cold_side/1(Heat_rate_Watt) -> [Heat_rate_cold_Watt]
  [air_properties_in_cold] -> Heat_load_cold_side/2(air_properties)
  [In_flow_bus_cold] -> Heat_load_cold_side/1(In_flow_bus)
  [Temp_cold_out_degreeC] -> Heat_load_cold_side/3(temp_out_degreeC)
  Heat_load_hot_side/1(Heat_rate_Watt) -> [Heat_rate_hot_Watt]
  [air_properties_in_hot] -> Heat_load_hot_side/2(air_properties)
  [In_flow_bus_hot] -> Heat_load_hot_side/1(In_flow_bus)
  [Temp_hot_out_degreeC] -> Heat_load_hot_side/3(temp_out_degreeC)
  [R_tot_KpW_cold] -> C_T_c_av/3(Tot_thermal_resist)
  [air_properties_in_cold] -> C_T_c_av/2(air_properties)
  [In_flow_bus_cold] -> C_T_c_av/1(In_flow_bus)
  C_T_c_av/1(C_T_c_av) -> [C_T_c_av]
  Re_number_in_cold/2(velo_air_ms-1) -> [v_in_mps_cold]
  Bus Creator2/1 -> Other_outputs/1
  Bus Creator1/1 -> Out_flow_bus_cold/1
  Bus Creator/1 -> Out_flow_bus_hot/1
  conservation _of_mass_cold_side/1 -> Bus Creator1/3  "mdot_kgps"
  Bus Selector3/1 -> conservation _of_mass_cold_side/1  "<mdot_kgps>"
  conservation _of_mass_hot_side/1 -> Bus Creator/3  "mdot_kgps"
  Bus Selector2/1 -> conservation _of_mass_hot_side/1  "<mdot_kgps>"
  [In_flow_bus_cold] -> Bus Selector3/1
  [In_flow_bus_hot] -> Bus Selector2/1
  [pres_Pa_out_cold] -> Pa to kPa1/1  "pres_Pa"
  [Temp_cold_out_degreeC] -> C to K1/1  "temp_C"
  [pres_Pa_out_hot] -> Pa to kPa/1  "pres_Pa"
  [Temp_hot_out_degreeC] -> C to K/1  "temp_C"
  Add2/1 -> [Temp_cold_out_degreeC]
  Add1/1 -> [Temp_hot_out_degreeC]
  Bus Selector1/1 -> Add2/1  "<temp_C>"
  Gain1/1 -> Add2/2
  Bus Selector/1 -> Add1/2  "<temp_C>"
  Gain/1 -> Add1/1
  [In_flow_bus_cold] -> Bus Selector1/1
  [In_flow_bus_hot] -> Bus Selector/1
  Calculating_T_h_av/1(T_h_av_degreC) -> Gain/1, [T_h_av_degreeC]
  Calculating_T_c_av/1(T_c_av_degreC) -> Gain1/1, [T_c_av_degreeC]
  [C_T_c_av] -> Calculating_T_c_av/3(C_t_c_av)
  [In_flow_bus_cold] -> Calculating_T_c_av/2(In_flow_bus)
  [Core_mass_temp_C] -> Calculating_T_c_av/1(T_cm)
  [C_T_h_av] -> Calculating_T_h_av/3(C_t_h_av)
  C_T_h_av/1(C_T_h_av) -> [C_T_h_av]
  [In_flow_bus_hot] -> Calculating_T_h_av/2(In_flow_bus)
  [Core_mass_temp_C] -> Calculating_T_h_av/1(T_cm)
  Calculating_core_mass_temp/1(Core_mass_temp_C) -> [Core_mass_temp_C]
  [R_tot_KpW_hot] -> C_T_h_av/3(Tot_thermal_resist)
  [air_properties_in_hot] -> C_T_h_av/2(air_properties)
  [In_flow_bus_hot] -> C_T_h_av/1(In_flow_bus)
  [In_flow_bus_cold] -> Calculating_core_mass_temp/5(In_flow_bus_cold)
  [In_flow_bus_hot] -> Calculating_core_mass_temp/4(In_flow_bus_hot)
  C_T_cm/1 -> Calculating_core_mass_temp/3(C_t_cm)
  C_T_c_i/1(C_T_c_i) -> Calculating_core_mass_temp/2(C_T_c_i), C_T_cm/2
  C_T_h_i/1(C_T_h_i) -> Calculating_core_mass_temp/1(C_T_h_i), C_T_cm/1
  [HX_parameters] -> C_T_c_i/4(HX_parameters)
  [R_tot_KpW_cold] -> C_T_c_i/3(Tot_thermal_resist)
  [air_properties_in_cold] -> C_T_c_i/2(air_properties)
  [In_flow_bus_cold] -> C_T_c_i/1(In_flow_bus)
  [HX_parameters] -> C_T_h_i/4(HX_parameters)
  [R_tot_KpW_hot] -> C_T_h_i/3(Tot_thermal_resist)
  Thermal_resistance_KpW_cold/1(R_tot_K/W) -> [R_tot_KpW_cold]
  Thermal_resistance_KpW_hot/1(R_tot_K/W) -> [R_tot_KpW_hot]
  [air_properties_in_hot] -> C_T_h_i/2(air_properties)
  [In_flow_bus_hot] -> C_T_h_i/1(In_flow_bus)
  [HX_parameters] -> Thermal_resistance_KpW_cold/2(HX_parameters)
  [Fin_parameters] -> Thermal_resistance_KpW_cold/3(Fin_parameters)
  [HTC_Wpm2K_cold] -> Thermal_resistance_KpW_cold/1(Convective_HTC)
  [HX_parameters] -> Thermal_resistance_KpW_hot/2(HX_parameters)
  [Fin_parameters] -> Thermal_resistance_KpW_hot/3(Fin_parameters)
  [HTC_Wpm2K_hot] -> Thermal_resistance_KpW_hot/1(Convective_HTC)
  convective_HTC_Wm-2K-1_cold/1(Convective_HTC_Wm-2K-1) -> [HTC_Wpm2K_cold]
  convective_HTC_Wm-2K-1_hot/1(Convective_HTC_Wm-2K-1) -> [HTC_Wpm2K_hot]
  Pressure_drop_cold/2(pres_Pa) -> [pres_Pa_out_cold]
  Pressure_drop_hot/2(pres_Pa) -> [pres_Pa_out_hot]
  Pressure_drop_cold/1(pres_drop_Pa) -> [delta_pres_Pa_cold]
  Pressure_drop_hot/1(pres_drop_Pa) -> [delta_pres_Pa_hot]
  Colburn_J_factor_cold/1(Colburn_J_factor) -> convective_HTC_Wm-2K-1_cold/1(Colburn_J_factor), [Colburn_J_factor_cold]
  [Hydraulic_diam_m] -> convective_HTC_Wm-2K-1_cold/4(hydraulic_diameter)
  [air_properties_in_cold] -> convective_HTC_Wm-2K-1_cold/3(air_properties)
  [Re_number_in_cold] -> convective_HTC_Wm-2K-1_cold/2(Re)
  [Hydraulic_diam_m] -> convective_HTC_Wm-2K-1_hot/4(hydraulic_diameter)
  [air_properties_in_hot] -> convective_HTC_Wm-2K-1_hot/3(air_properties)
  [Re_number_in_hot] -> convective_HTC_Wm-2K-1_hot/2(Re)
  Colburn_J_factor_hot/1(Colburn_J_factor) -> convective_HTC_Wm-2K-1_hot/1(Colburn_J_factor), [Colburn_J_factor_hot]
  Friction_factor_cold/1(Friction_factor) -> Pressure_drop_cold/1(Friction_factor), [Fricn_factor_cold]
  [In_flow_bus_cold] -> Pressure_drop_cold/6(In_flow_bus)
  [Hydraulic_diam_m] -> Pressure_drop_cold/5(D_hydraulic)
  [v_in_mps_cold] -> Pressure_drop_cold/4(air_velocity)
  [air_properties_in_cold] -> Pressure_drop_cold/3(air_properties)
  [HX_parameters] -> Pressure_drop_cold/2(HX_parameters)
  [In_flow_bus_hot] -> Pressure_drop_hot/6(In_flow_bus)
  Friction_factor_hot/1(Friction_factor) -> Pressure_drop_hot/1(Friction_factor), [Fricn_factor_hot]
  [Hydraulic_diam_m] -> Pressure_drop_hot/5(D_hydraulic)
  [v_in_mps_hot] -> Pressure_drop_hot/4(air_velocity)
  [air_properties_in_hot] -> Pressure_drop_hot/3(air_properties)
  [HX_parameters] -> Pressure_drop_hot/2(HX_parameters)
  Re_number_in_hot/2(velo_air_ms-1) -> [v_in_mps_hot]
  [Re_number_in_cold] -> Colburn_J_factor_cold/2(Re)
  [Fin_parameters_ratios] -> Colburn_J_factor_cold/1(Fin_prameter_ratios)
  [Re_number_in_cold] -> Friction_factor_cold/2(Re)
  [Fin_parameters_ratios] -> Friction_factor_cold/1(Fin_prameter_ratios)
  [Re_number_in_hot] -> Colburn_J_factor_hot/2(Re)
  [Fin_parameters_ratios] -> Colburn_J_factor_hot/1(Fin_prameter_ratios)
  [Re_number_in_hot] -> Friction_factor_hot/2(Re)
  [Fin_parameters_ratios] -> Friction_factor_hot/1(Fin_prameter_ratios)
  HX_and_Fin_paramters/3(Fin_parameters_ratios) -> [Fin_parameters_ratios]
  [air_properties_in_cold] -> Re_number_in_cold/2(air_properties)
  [In_flow_bus_cold] -> Re_number_in_cold/1(In_flow_bus)
  [HX_parameters] -> Re_number_in_cold/4(HX_paramters), Re_number_in_hot/4(HX_paramters)
  [Hydraulic_diam_m] -> Re_number_in_cold/3(Hydraulic_diam), Re_number_in_hot/3(Hydraulic_diam)
  [air_properties_in_hot] -> Re_number_in_hot/2(air_properties)
  [In_flow_bus_hot] -> Re_number_in_hot/1(In_flow_bus)
  [In_flow_bus_cold] -> Air_properties_in_flows_hot_and_cold/2(In_flow_bus_cold)
  [In_flow_bus_hot] -> Air_properties_in_flows_hot_and_cold/1(In_flow_bus_hot)
  Air_properties_in_flows_hot_and_cold/2(air_properties_in_cold1) -> [air_properties_in_cold]
  Air_properties_in_flows_hot_and_cold/1(air_properties_in_hot1) -> [air_properties_in_hot]
  HX_and_Fin_paramters/2(Fin_parameters1) -> [Fin_parameters]
  HX_and_Fin_paramters/1(HX_parameters2) -> [HX_parameters]
  Re_number_in_cold/1(Re_number) -> [Re_number_in_cold]
  Re_number_in_hot/1(Re_number) -> [Re_number_in_hot]
  Hydraulic_diam_m/1(Out1) -> [Hydraulic_diam_m]
  [Fin_parameters] -> Hydraulic_diam_m/1(Fin_parameters)
  C to K/1 -> Bus Creator/1  "temp_K"
  Pa to kPa/1 -> Bus Creator/2  "pres_kPa"
  C to K1/1 -> Bus Creator1/1  "temp_K"
  Pa to kPa1/1 -> Bus Creator1/2  "pres_kPa"
  [Heat_rate_cold_Watt] -> Bus Creator2/13  "Heat_rate_cold_Watt"
  [Heat_rate_hot_Watt] -> Bus Creator2/12  "Heat_rate_hot_Watt"
  [Core_mass_temp_C] -> Bus Creator2/11  "HX_core_mass_temp_C"
  [Fricn_factor_hot] -> Bus Creator2/3  "f_hot"
  [Fricn_factor_cold] -> Bus Creator2/4  "f_cold"
  [Colburn_J_factor_hot] -> Bus Creator2/5  "J_hot"
  [Colburn_J_factor_cold] -> Bus Creator2/6  "J_cold"
  [HTC_Wpm2K_hot] -> Bus Creator2/7  "h_hot"
  [HTC_Wpm2K_cold] -> Bus Creator2/8  "h_cold"
  [delta_pres_Pa_hot] -> Bus Creator2/9  "Delta_P_hot"
  [delta_pres_Pa_cold] -> Bus Creator2/10  "Delta_P_cold"
  [Re_number_in_hot] -> Bus Creator2/1  "Re_hot"
  [Re_number_in_cold] -> Bus Creator2/2  "Re_cold"
  In_flow_bus_hot/1 -> Bus Selector4/1
  Bus Selector4/1 -> Bus Creator3/1  "<mdot_kgps>"
  Bus Selector4/2 -> K to C/1  "<temp_K>"
  Bus Selector4/3 -> kPa to Pa/1  "<pres_kPa>"
  K to C/1 -> Bus Creator3/2  "temp_C"
  Bus Creator3/1 -> [In_flow_bus_hot]
  kPa to Pa/1 -> Bus Creator3/3  "pres_Pa"
  Bus Selector5/1 -> Bus Creator4/1  "<mdot_kgps>"
  Bus Selector5/2 -> K to C1/1  "<temp_K>"
  Bus Selector5/3 -> kPa to Pa1/1  "<pres_kPa>"
  K to C1/1 -> Bus Creator4/2  "temp_C"
  kPa to Pa1/1 -> Bus Creator4/3  "press_Pa"
  Bus Creator4/1 -> [In_flow_bus_cold]
  [T_h_av_degreeC] -> Bus Creator2/14  "T_av_hot_C"
  [T_c_av_degreeC] -> Bus Creator2/15  "T_av_cold_C"
  In_flow_bus_cold/1 -> Bus Selector5/1
